simulink library "raspi_library"  (R2017a)
settings: Solver=VariableStepAuto  StartTime=0.0  StopTime=10.0  RelTol=1e-3
undefined symbols (not defined in the file or in its folder): H, prms
libraries: simulink x3, raspi_library x1
settings Model: Creator=marti  LastModifiedBy=marti

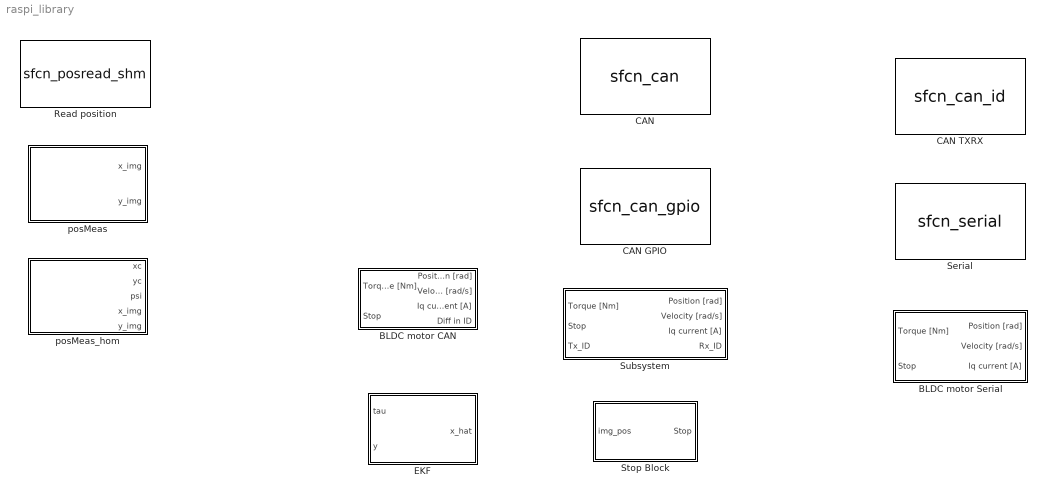
== system raspi_library ==
  BLDC motor CAN : Subsystem  mask{sampleTime=prms.Ts}
      mask prompts: sampleTime "Sampling Time"
  BLDC motor Serial : Subsystem  mask{sampleTime=prms.Ts}
      mask prompts: sampleTime "Sampling time"
  CAN : S-Function  InitFcn=try, set_param(gcb,'FunctionName','sfcn_can'), end  FunctionName=sfcn_can  Parameters=sampleTime  SFunctionModules=sfcn_can_wrapper  SFunctionDeploymentMode=off  EnableBusSupport=off  mask(S-Function Builder){}
      mask init:
      | val = [[.9  0.75 0.75 1 1 .9 .9 1]',[1 1 0.75 0.75 .9 .9 1 .9]'];try , sys = get_param(gcb,'SfunBuilderFcnName');if isempty(sys), sys = get_param(gcb,'FunctionName'); end,catch, sys = get_param(gcb,'FunctionName'); end
      settings: CopyFcn=set_param(gcbh,'LinkStatus','none')  PreSaveFcn=try, set_param(gcb,'FunctionName','sfcn_can'), end  OpenFcn=sfunctionwizard(gcbh)
      mask Display: plot(val(:,1),val(:,2)),disp(sys), port_label('input',1,'in'), port_label('output',1,'pos'), port_label('output',2,'vel'), port_label('output',3,'iq')
  CAN GPIO : S-Function  InitFcn=try, set_param(gcb,'FunctionName','sfcn_can_gpio'), end  FunctionName=sfcn_can_gpio  Parameters=sampleTime  SFunctionModules=sfcn_can_gpio_wrapper  SFunctionDeploymentMode=off  EnableBusSupport=off  mask(S-Function Builder){}
      mask init: same as raspi_library/CAN
      settings: CopyFcn=set_param(gcbh,'LinkStatus','none')  PreSaveFcn=try, set_param(gcb,'FunctionName','sfcn_can_gpio'), end  OpenFcn=sfunctionwizard(gcbh)
      mask Display: plot(val(:,1),val(:,2)),disp(sys), port_label('input',1,'in'), port_label('output',1,'pos'), port_label('output',2,'vel'), port_label('output',3,'iq')
  CAN TXRX : S-Function  InitFcn=try, set_param(gcb,'FunctionName','sfcn_can_id'), end  FunctionName=sfcn_can_id  Parameters=sampleTime  SFunctionModules=sfcn_can_id_wrapper  SFunctionDeploymentMode=off  EnableBusSupport=off  mask(S-Function Builder){}
      mask init: same as raspi_library/CAN
      settings: CopyFcn=set_param(gcbh,'LinkStatus','none')  PreSaveFcn=try, set_param(gcb,'FunctionName','sfcn_can_id'), end  OpenFcn=sfunctionwizard(gcbh)
      mask Display: plot(val(:,1),val(:,2)),disp(sys), port_label('input',1,'in'), port_label('input',2,'tx_id'), port_label('output',1,'pos'), port_label('output',2,'vel'), port_label('output',3,'iq'), port_label('output',4,'rx_id')
  EKF : Subsystem
  Read position : S-Function  InitFcn=try, set_param(gcb,'FunctionName','sfcn_posread_shm'), end  FunctionName=sfcn_posread_shm  Parameters=sampleTime  SFunctionModules=sfcn_posread_shm_wrapper  SFunctionDeploymentMode=off  EnableBusSupport=off  mask(S-Function Builder){}
      mask init: same as raspi_library/CAN
      settings: CopyFcn=set_param(gcbh,'LinkStatus','none')  PreSaveFcn=try, set_param(gcb,'FunctionName','sfcn_posread_shm'), end  OpenFcn=sfunctionwizard(gcbh)
      mask Display: plot(val(:,1),val(:,2)),disp(sys), port_label('output',1,'pos_x'), port_label('output',2,'pos_y')
  Serial : S-Function  InitFcn=try, set_param(gcb,'FunctionName','sfcn_serial'), end  FunctionName=sfcn_serial  Parameters=1  SFunctionModules=sfcn_serial_wrapper  SFunctionDeploymentMode=off  EnableBusSupport=off  mask(S-Function Builder){}
      mask init: same as raspi_library/CAN
      settings: CopyFcn=set_param(gcbh,'LinkStatus','none')  PreSaveFcn=try, set_param(gcb,'FunctionName','sfcn_serial'), end  OpenFcn=sfunctionwizard(gcbh)
      mask Display: plot(val(:,1),val(:,2)),disp(sys), port_label('input',1,'in'), port_label('output',1,'pos'), port_label('output',2,'vel'), port_label('output',3,'iq')
  Stop Block : Subsystem
  Subsystem : Subsystem  mask{sampleTime=prms.Ts}
      mask prompts: sampleTime "Sampling Time"
  posMeas : Subsystem  mask{sampleTime=1/50}
      mask prompts: sampleTime "Sampling time"
  posMeas_hom : Subsystem  InitFcn=|  mask{H=H, sampleTime=prms.Ts}
      | %simul_time = str2num(get_param(gcs, 'StopTime'));
      | %fps = 50;
      | %num_frames = round(50*(simul_time+30));
      | %stream = 0;
      | %exposition_time = 5;
      | 
      | %if ~exist('mypi')
      | % mypi = raspi(ip_rpi, rpi_user, rpi_passwd);
      | %end
      | % run the script measuring the position on raspi
      | %rpi_posMes_run( mypi, fps, num_frames, stream, exposition_time )
      mask prompts: H "Calibration Matrix"; sampleTime "Sampling Time"

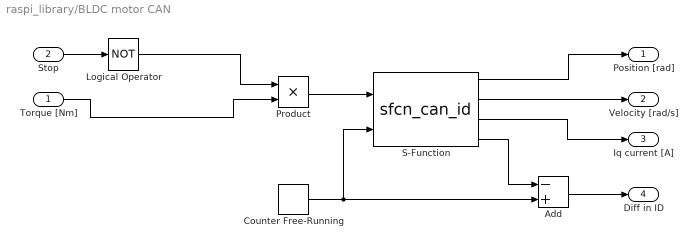
== system raspi_library/BLDC motor CAN ==
  Torque [Nm] : Inport  OutDataTypeStr=single
  Stop : Inport  Port=2  OutDataTypeStr=boolean
  Add : Sum  Inputs=-+  OutDataTypeStr=uint32
  Counter Free-Running : simulink/Sources/Counter Free-Running  NumBits=32  tsamp=sampleTime
  Logical Operator : Logic  Operator=NOT  AllPortsSameDT=off  OutDataTypeStr=boolean
  Product : Product
  S-Function : S-Function  FunctionName=sfcn_can_id  Parameters=sampleTime  SFunctionModules=sfcn_can_id_wrapper  SFunctionDeploymentMode=off  EnableBusSupport=off
  Position [rad] : Outport  OutDataTypeStr=single
  Velocity [rad/s] : Outport  Port=2  OutDataTypeStr=single
  Iq current [A] : Outport  Port=3  OutDataTypeStr=single
  Diff in ID : Outport  Port=4  OutDataTypeStr=uint32
  wires:
  S-Function/3 -> Iq current [A]/1
  Torque [Nm]/1 -> Product/2
  Product/1 -> S-Function/1
  Stop/1 -> Logical Operator/1
  Logical Operator/1 -> Product/1
  S-Function/2 -> Velocity [rad/s]/1
  S-Function/1 -> Position [rad]/1
  Counter Free-Running/1 -> S-Function/2, Add/2
  S-Function/4 -> Add/1
  Add/1 -> Diff in ID/1

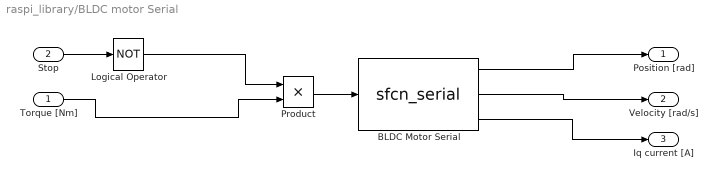
== system raspi_library/BLDC motor Serial ==
  Torque [Nm] : Inport
  Stop : Inport  Port=2
  BLDC Motor Serial : S-Function  FunctionName=sfcn_serial  Parameters=sampleTime  SFunctionModules=sfcn_serial_wrapper  SFunctionDeploymentMode=off  EnableBusSupport=off
  Logical Operator : Logic  Operator=NOT  AllPortsSameDT=off  OutDataTypeStr=boolean
  Product : Product
  Position [rad] : Outport
  Velocity [rad/s] : Outport  Port=2
  Iq current [A] : Outport  Port=3
  wires:
  BLDC Motor Serial/2 -> Velocity [rad/s]/1
  Product/1 -> BLDC Motor Serial/1
  BLDC Motor Serial/1 -> Position [rad]/1
  Logical Operator/1 -> Product/1
  BLDC Motor Serial/3 -> Iq current [A]/1
  Stop/1 -> Logical Operator/1
  Torque [Nm]/1 -> Product/2

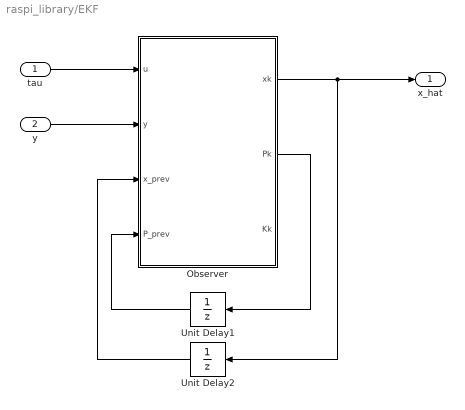
== system raspi_library/EKF ==
  tau : Inport  OutDataTypeStr=single
  y : Inport  Port=2  OutDataTypeStr=single
  Observer : MATLAB Function  TreatAsAtomicUnit=on  SystemSampleTime=prms.Ts
  Unit Delay1 : UnitDelay  InitialCondition=prms.out.P0  SampleTime=prms.Ts
  Unit Delay2 : UnitDelay  InitialCondition=prms.out.x0  SampleTime=prms.Ts
  x_hat : Outport  OutDataTypeStr=single
  wires:
  Unit Delay2/1 -> Observer/3(x_prev)
  Observer/2(Pk) -> Unit Delay1/1
  Unit Delay1/1 -> Observer/4(P_prev)
  Observer/1(xk) -> x_hat/1, Unit Delay2/1
  tau/1 -> Observer/1(u)
  y/1 -> Observer/2(y)

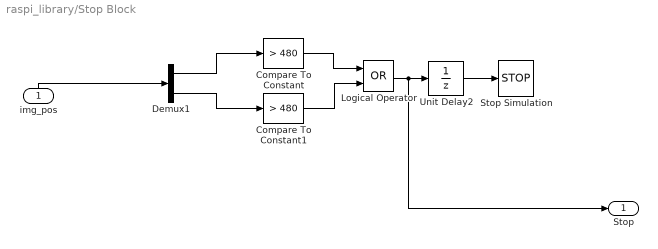
== system raspi_library/Stop Block ==
  img_pos : Inport
  Compare To Constant : simulink/Logic and Bit Operations/Compare To Constant  relop=>  const=480  OutDataTypeStr=boolean
  Compare To Constant1 : simulink/Logic and Bit Operations/Compare To Constant  relop=>  const=480  OutDataTypeStr=boolean
  Demux1 : Demux  Outputs=2
  Logical Operator : Logic  Operator=OR  AllPortsSameDT=off  OutDataTypeStr=boolean
  Stop Simulation : Stop
  Unit Delay2 : UnitDelay  SampleTime=prms.Ts
  Stop : Outport
  wires:
  Unit Delay2/1 -> Stop Simulation/1
  img_pos/1 -> Demux1/1
  Logical Operator/1 -> Stop/1, Unit Delay2/1
  Demux1/2 -> Compare To Constant1/1
  Compare To Constant/1 -> Logical Operator/1
  Demux1/1 -> Compare To Constant/1
  Compare To Constant1/1 -> Logical Operator/2

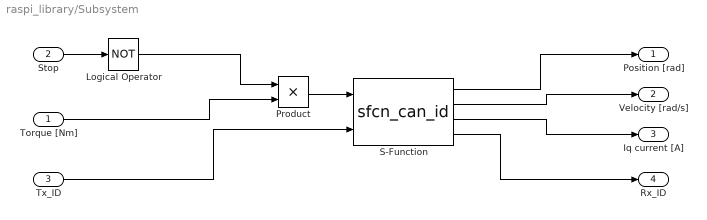
== system raspi_library/Subsystem ==
  Torque [Nm] : Inport
  Stop : Inport  Port=2
  Tx_ID : Inport  Port=3
  Logical Operator : Logic  Operator=NOT  AllPortsSameDT=off  OutDataTypeStr=boolean
  Product : Product
  S-Function : S-Function  FunctionName=sfcn_can_id  Parameters=sampleTime  SFunctionModules=sfcn_can_id_wrapper  SFunctionDeploymentMode=off  EnableBusSupport=off
  Position [rad] : Outport
  Velocity [rad/s] : Outport  Port=2
  Iq current [A] : Outport  Port=3
  Rx_ID : Outport  Port=4
  wires:
  Torque [Nm]/1 -> Product/2
  Logical Operator/1 -> Product/1
  Product/1 -> S-Function/1
  S-Function/1 -> Position [rad]/1
  S-Function/3 -> Iq current [A]/1
  Stop/1 -> Logical Operator/1
  Tx_ID/1 -> S-Function/2
  S-Function/2 -> Velocity [rad/s]/1
  S-Function/4 -> Rx_ID/1

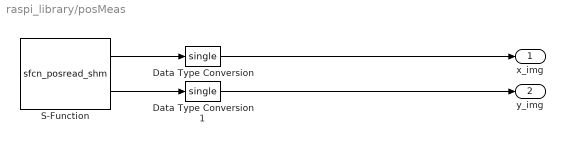
== system raspi_library/posMeas ==
  Data Type Conversion : DataTypeConversion  OutDataTypeStr=single
  Data Type Conversion1 : DataTypeConversion  OutDataTypeStr=single
  S-Function : S-Function  FunctionName=sfcn_posread_shm  Parameters=sampleTime  SFunctionModules=sfcn_posread_shm_wrapper  SFunctionDeploymentMode=off  EnableBusSupport=off
  x_img : Outport
  y_img : Outport  Port=2
  wires:
  S-Function/2 -> Data Type Conversion1/1
  Data Type Conversion1/1 -> y_img/1
  Data Type Conversion/1 -> x_img/1
  S-Function/1 -> Data Type Conversion/1

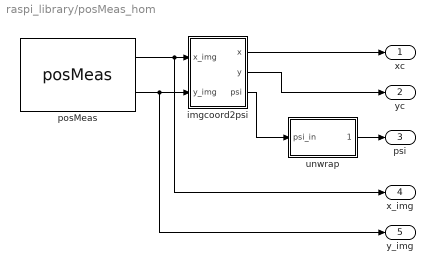
== system raspi_library/posMeas_hom ==
  imgcoord2psi : Subsystem
  posMeas : raspi_library/posMeas  sampleTime=sampleTime
  unwrap : Subsystem
  xc : Outport
  yc : Outport  Port=2
  psi : Outport  Port=3
  x_img : Outport  Port=4
  y_img : Outport  Port=5
  wires:
  posMeas/1 -> x_img/1, imgcoord2psi/1(x_img)
  posMeas/2 -> y_img/1, imgcoord2psi/2(y_img)
  imgcoord2psi/3(psi) -> unwrap/1(psi_in)
  unwrap/1(psi_out) -> psi/1
  imgcoord2psi/1(x) -> xc/1
  imgcoord2psi/2(y) -> yc/1

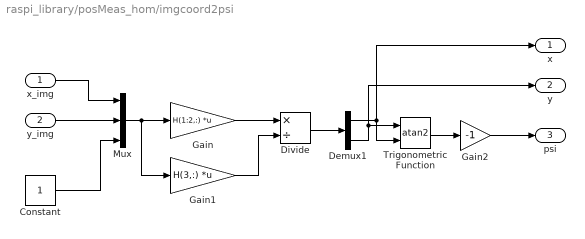
== system raspi_library/posMeas_hom/imgcoord2psi ==
  x_img : Inport
  y_img : Inport  Port=2
  Constant : Constant  OutDataTypeStr=single
  Demux1 : Demux  Outputs=2
  Divide : Product  Inputs=*/
  Gain : Gain  Gain=H(1:2,:)  Multiplication=Matrix(K*u)
  Gain1 : Gain  Gain=H(3,:)  Multiplication=Matrix(K*u)
  Gain2 : Gain  Gain=-1  OutDataTypeStr=single
  Mux : Mux  Inputs=3
  Trigonometric Function : Trigonometry  Operator=atan2  OutputSignalType=real
  x : Outport
  y : Outport  Port=2
  psi : Outport  Port=3
  wires:
  Mux/1 -> Gain1/1, Gain/1
  Constant/1 -> Mux/3
  Demux1/2 -> y/1, Trigonometric Function/1
  Gain/1 -> Divide/1
  Gain1/1 -> Divide/2
  Divide/1 -> Demux1/1
  Demux1/1 -> x/1, Trigonometric Function/2
  x_img/1 -> Mux/1
  y_img/1 -> Mux/2
  Trigonometric Function/1 -> Gain2/1
  Gain2/1 -> psi/1

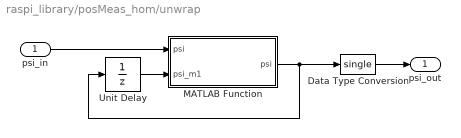
== system raspi_library/posMeas_hom/unwrap ==
  psi_in : Inport
  Data Type Conversion : DataTypeConversion  OutDataTypeStr=single
  MATLAB Function : MATLAB Function  TreatAsAtomicUnit=on
  Unit Delay : UnitDelay  InitialCondition=single(0)  SampleTime=prms.Ts
  psi_out : Outport
  wires:
  MATLAB Function/1(psi) -> Data Type Conversion/1, Unit Delay/1
  Unit Delay/1 -> MATLAB Function/2(psi_m1)
  psi_in/1 -> MATLAB Function/1("psi ")
  Data Type Conversion/1 -> psi_out/1

== matlab function raspi_library/EKF/Observer ==
  settings: updateMethod=DISCRETE  sampleTime=prms.Ts
  data: u input; y input; xk output single; x_prev input; P_prev input; Pk output; Kk output; prms parameter
function [xk, Pk, Kk] = EKF( u, y, x_prev, P_prev, prms)

Q =  prms.out.KF.Q;
R =  prms.out.KF.R;
% R = R([1 3], [1 3]);
% y = y([1 3]);

[Ak_c, ~, Hk, ~] = ballInAHoopODEFUN_linMatrices(x_prev, u, prms);
% Hk = Hk([1 3],:);
Ak = eye(size(P_prev)) + prms.Ts*Ak_c; % discretized version of the system matrix

% Time Update
xk = x_prev + prms.Ts*ballInAHoopODEFUN(0, x_prev, prms, u);
Pk = Ak*P_prev*Ak'+Q;

% Measurement Update
Kk = Pk*Hk'/(Hk*Pk*Hk'+R);
xk = xk + Kk*(y-Hk*xk);
Pk = (eye(size(P_prev))-Kk*Hk)*Pk;

== matlab function raspi_library/posMeas_hom/unwrap/MATLAB Function ==
  data: psi input; psi output; psi_m1 input
function psi = unwrap(psi, psi_m1)
%%% The code is taken from the Matlab function unwrap

% Unwrap phase angles.  Algorithm minimizes the incremental phase variation 
% by constraining it to the range [-pi,pi]
dp = psi - psi_m1;                % Incremental phase variations

% Compute an integer describing how many times 2*pi we are off:
% dp in [-pi, pi]: dp_corr = 0,
% elseif dp in [-3*pi, 3*pi]: dp_corr = 1,
% else if dp in [-5*pi, 5*pi]: dp_corr = 2, ...
dp_corr = dp./(2*pi);

% We want to do round(dp_corr), except that we want the tie-break at n+0.5
% to round towards zero instead of away from zero (that is, (2n+1)*pi will
% be shifted by 2n*pi, not by (2n+2)*pi):
roundDown = abs(rem(dp_corr, 1)) <= 0.5;
dp_corr(roundDown) = fix(dp_corr(roundDown));

dp_corr = round(dp_corr);

% Stop the jump from happening if dp < cutoff (no effect if cutoff <= pi)
dp_corr(abs(dp) < pi) = 0;

% Integrate corrections and add to P to produce smoothed phase values
psi = single(psi - (2*pi)*cumsum(dp_corr,1));
